simulink model "test00_mdl"  (R2024a)
settings: Solver=ode1  StartTime=0.0  StopTime=Inf  FixedStep=0.001  RelTol=1e-3
PostLoadFcn:
  | , if any(exist('dsrtsu_mdlpostloadfcn', 'file') ~= 0), dsrtsu_mdlpostloadfcn('Execute', bdroot); end,
InitFcn:
  | , if any(exist('rtifpga_mdlclblib', 'file') ~= 0), rtifpga_mdlclblib('Init', bdroot); end,
libraries: rti1401lib_dio_type3 x2, rti1401lib_adc_type4 x1, rti1401lib_II_base x1
Description:
  | Standard RTI1401 template.
  | Supported MATLAB version:  R2024a.
settings Model: Tag=RTI1401  DSRTSU_INTERNAL_RTI_VER=640  DSRTSU_INTERNAL_RTI_TYPE=rti1401  RTICANMMDATA=struct('GeneralSetupData',struct('modelroot','C:\Users\VM-User\Desktop\MigrationScripts','generalsettings',struct('filesettings',struct('destfolder',struct('Name','RTICANMM_FILES','Check',1),'buildfolder',struct('Name','.','Check',1),'AbsDestfolder',struct('Name','C:\Users\VM-User\Desktop\MigrationScripts\RTICANMM_FILES'),'AbsBuildfolder',struct('Name','C:\Users\VM-User\Desktop\MigrationScripts'))),'options',struct('addpaths',1,'rmpaths',1,'addtrcexclusion',true,'cannavigator',struct('checkmonitoring',0),'show_usrtrc',0,'use_usrtrc',0),'advanced',struct('options',ones(1,100)),'MPSetup',{{}},'RTI',struct('Type','RTI1401','Ver','7.17','Date','02-Nov-2021'),'modelname','','block','untitled'))  DSRTSU_INTERNAL_RTIFPGA=210  DSRTSU_INTERNAL_RTISTBM_VER=24.1  Creator=carpc  LastModifiedBy=carpc
settings SolverCC: AlgebraicLoopSolver=TrustRegion
settings DataIOCC: ReturnWorkspaceOutputs=off
settings OptimizationCC: BlockReduction=off  OptimizeBlockIOStorage=off  BufferReuse=off  ReuseModelBlockBuffer=off  GlobalBufferReuse=off  ExpressionFolding=off  LocalBlockOutputs=off  OptimizeDataStoreBuffers=off  BusAssignmentInplaceUpdate=off
settings DebuggingCC: UnconnectedInputMsg=warning  UnconnectedOutputMsg=warning  UnconnectedLineMsg=warning  PregeneratedLibrarySubsystemCodeDiagnostic=none  ArithmeticOperatorsInVariantConditions=warning
settings HardwareCC: ProdBitPerPointer=32  ProdBitPerSizeT=32  ProdBitPerPtrDiffT=32  ProdLargestAtomicInteger=Integer  ProdEndianess=BigEndian  ProdWordSize=32  ProdLongLongMode=on  ProdHWDeviceType=Custom Processor->Custom  TargetIntDivRoundTo=Zero  TargetEndianess=BigEndian  TargetHWDeviceType=Custom Processor->Custom
settings ModelReferenceCC: EnableRefExpFcnMdlSchedulingChecks=on  EnableParallelModelReferenceBuilds=on  ParallelModelReferenceMATLABWorkerInit=Load Top Model
settings SFSimCC: SimUseLocalCustomCode=off  MATLABDynamicMemAlloc=off  CustomCodeUndefinedFunction=UseInterfaceOnly
settings RTWCC: Description=dSPACE DS1401 Hardware Platform  SystemTargetFile=rti1401.tlc  MakeCommand=make_rti  TemplateMakefile=rti1401.tmf  RTWUseLocalCustomCode=off  GPUComputeCapability=3.5  DLArmComputeVersion=19.05
settings CodeAppCC: StateflowObjectComments=on
settings STFCustomTargetCC: TargetLangStandard=C89/C90 (ANSI)  ParMdlRefBuildCompliant=on  GRTInterface=off  UseToolchainInfoCompliant=off  SystemTargetFile=rti1401.tlc
settings GRTTargetCC: TargetLangStandard=C89/C90 (ANSI)  CompOptLevelCompliant=off  ConcurrentExecutionCompliant=off  CombineOutputUpdateFcns=off  MatFileLogging=off  CPPClassGenCompliant=off  UseToolchainInfoCompliant=off
settings ConfigComp: CovMetricSettings=dswe

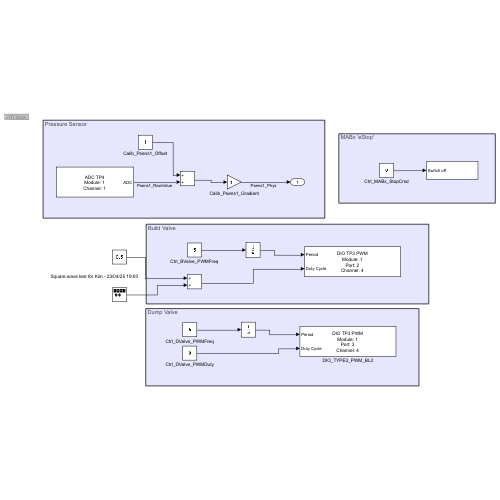
[thumbnail: Simulink's stored preview of the top-level diagram]
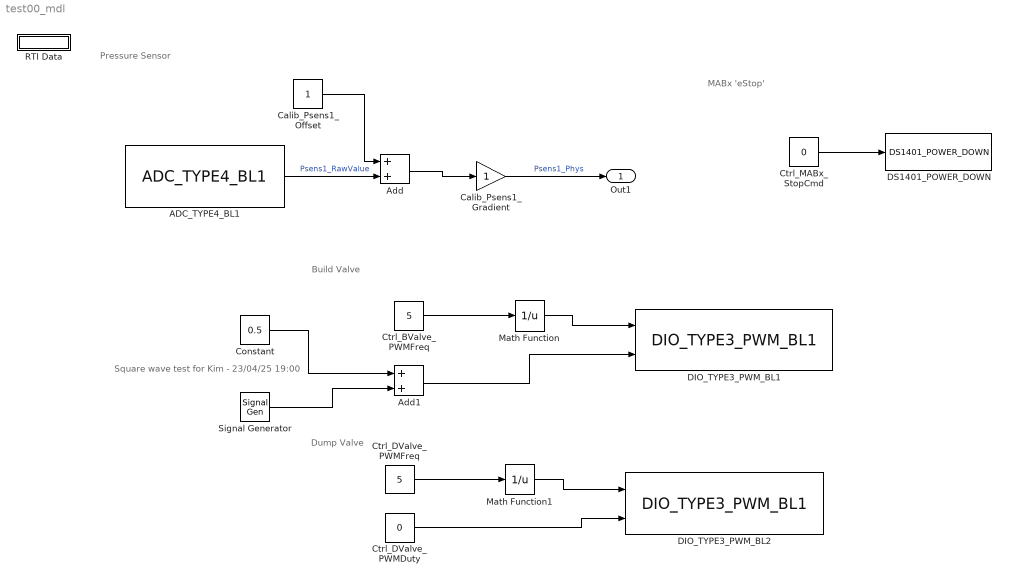
== system test00_mdl ==
  note: Square wave test for Kim - 23/04/25 19:00
  note: MABx 'eStop'
  note: Pressure Sensor
  note: Build Valve
  note: Dump Valve
  ADC_TYPE4_BL1 : rti1401lib_adc_type4/ADC_TYPE4_BL1  DSProperties=struct('RTI',struct('Version',uint32(2),'BlockType',struct('isSLSource',uint8(1),'isSLSink',uint8(1),'isHWSource',uint8(0),'isHWSink',uint8(1),'isSetup',uint8(0),'isInline',uint8(1),'isNonInline',uint8(0),'isInterrupt',uint8(0),'isChannelwise',uint8(1)),'IOBoardType',{{'DS1401','STD','ADCT4'}},'UnitType','ADC','Identifier','ADC','DialogType','ML','BlockSet','NONE','SlaveProcessor','NONE'))  RTIBlockInterface=struct('InputPortsActive',0,'InputPortsWidth',int32(1),'InputPortsDataType',{{'SS_BOOLEAN'}},'InputPortsName',{{'Continue'}},'OutputPortsActive',[1 0],'OutputPortsWidth',int32([1 1]),'OutputPortsDataType',{{'SS_DOUBLE','SS_UINT8'}},'OutputPortsName',{{'ADC','Status'}},'DialogFcn','rti1401stdadct4adcgui','SampleTime',{{-1}},'InitLevel',3,'IconTransparency','on','BlockDisplay',{{['ADC TP4\nModule: 1\nChannel: 1'],'center'}},'BlockName',struct('Token',{{'ADC_TYPE4_BL1'}}))  RTIBlockParameters=struct('ADCSWStartDisable',{{0,'OFF',[0 1]}},'ModuleNo',{{1,'OFF',[1 16]}},'ChannelNo',{{1,'OFF',[1 16]}},'ConversionMode',{{1,'OFF',[1 2]}},'SampleMode',{{1,'OFF',[1 2]}},'TriggerSource',{{1,'OFF',[1 5]}},'EdgePolarity',{{1,'OFF',[1 2]}},'ConversionTriggerSource',{{2,'OFF',[1 6]}},'ConversionEdgePolarity',{{1,'OFF',[1 2]}},'ConversionPeriod',{{1e-6,'OFF',[]}},'ConversionPeriodCheck',{{0,'OFF',[]}},'BurstTriggerSource',{{1,'OFF',[1 6]}},'BurstEdgePolarity',{{1,'OFF',[1 2]}},'BurstSize',{{10,'OFF',[]}},'BurstSizeCheck',{{0,'OFF',[]}},'DataSetOffset',{{0,'OFF',[]}},'DataSetOffsetCheck',{{0,'OFF',[]}},'DataSetLength',{{1,'OFF',[]}},'DataSetLengthCheck',{{0,'OFF',[]}},'ReadMode',{{1,'OFF',[1 2]}},'SampleTime',{{-1,'OFF',[-1 inf]}},'SampleTimeCheck',{{1,'OFF',[]}},'StatusPortEnable',{{0,'OFF',[0 1]}},'VoltageRange',{{1,'OFF',[1 2]}},'TLCFileName',{{'rti1401adc_t4_adc','OFF',[]}})  RTISFcnParameters=struct('ADCSWStartDisable','int32','ModuleNo','int32','ChannelNo','int16','ConversionMode','int16','SampleMode','int16','TriggerSource','int16','EdgePolarity','int16','ConversionTriggerSource','int16','ConversionEdgePolarity','int16','ConversionPeriod','double','BurstTriggerSource','int16','BurstEdgePolarity','int16','BurstSize','int16','DataSetOffset','int16','DataSetLength','int16','ReadMode','int16','SampleTime','double','StatusPortEnable','int16','VoltageRange','int16','TLCFileName','char')  RTIBlockParaDefault=struct('ADCSWStartDisable',0,'ModuleNo',1,'ChannelNo',1,'ConversionMode',1,'SampleMode',1,'TriggerSource',1,'EdgePolarity',1,'ConversionTriggerSource',2,'ConversionEdgePolarity',1,'ConversionPeriod',1e-6,'ConversionPeriodCheck',0,'BurstTriggerSource',1,'BurstEdgePolarity',1,'BurstSize',10,'BurstSizeCheck',0,'DataSetOffset',0,'DataSetOffsetCheck',0,'DataSetLength',1,'DataSetLengthCheck',0,'ReadMode',1,'SampleTime',-1,'SampleTimeCheck',1,'StatusPortEnable',0,'VoltageRange',1,'TLCFileName','rti1401adc_t4_adc')
  Add : Sum
  Add1 : Sum
  Calib_Psens1_Gradient : Gain
  Calib_Psens1_Offset : Constant
  Constant : Constant  Value=0.5
  Ctrl_BValve_PWMFreq : Constant  Value=5
  Ctrl_DValve_PWMDuty : Constant  Value=0
  Ctrl_DValve_PWMFreq : Constant  Value=5
  Ctrl_MABx_StopCmd : Constant  Value=0
  DIO_TYPE3_PWM_BL1 : rti1401lib_dio_type3/DIO_TYPE3_PWM_BL1  DSProperties=struct('RTI',struct('Version',uint32(2),'BlockType',struct('isSLSource',uint8(0),'isSLSink',uint8(1),'isHWSource',uint8(0),'isHWSink',uint8(1),'isSetup',uint8(0),'isInline',uint8(1),'isNonInline',uint8(0),'isInterrupt',uint8(0),'isChannelwise',uint8(1)),'IOBoardType',{{'DS1401','STD','DIOT3'}},'UnitType','PWM','Identifier','PWM','DialogType','ML','BlockSet','NONE','SlaveProcessor','NONE'))  RTIBlockInterface=struct('InputPortsWidth',int32([1 1]),'InputPortsActive',[1 1],'InputPortsName',{{'Period',['Duty Cycle']}},'BlockDisplay',{{['DIO TP3 PWM\nModule: 1\nPort: 2\nChannel: 4'],'center'}},'IconTransparency','on','InitLevel',3,'DialogFcn','rti1401stddiot3pwmgui','BlockName',struct('Token',{{'DIO_TYPE3_PWM_BL1'}}))  RTIBlockParameters=struct('ModuleNo',{{1,'OFF',[1 16]}},'PortNo',{{2,'OFF',[1 3]}},'ChannelNo',{{4,'OFF',[1 16]}},'SupplyRailsCh',{{[1 1],'OFF',[0 1 0 1]}},'UpdateMode',{{1,'ON',[1 2]}},'PeriodRange',{{7,'OFF',[1 16]}},'DutyCycleInit',{{'0','OFF',[0 1]}},'PeriodInit',{{'5e-05','OFF',[]}},'TerminationMode',{{0,'OFF',[0 1]}},'OutputTermValidate',{{0,'OFF',[0 1]}},'OutputTermBuildCheck',{{0,'OFF',[]}},'DutyCycleTerm',{{'0','OFF',[0 1]}},'PeriodTerm',{{'5e-05','OFF',[]}},'TLCFileName',{{'rti1401dio_t3_pwm','OFF',[]}},'EnableInterrupt',{{0,'OFF',[0 1]}},'TriggerEdgeType',{{1,'OFF',[1 3]}})  RTISFcnParameters=struct('ModuleNo','int32','PortNo','int16','ChannelNo','int16','SupplyRailsCh','int16','UpdateMode','int16','PeriodRange','int16','DutyCycleInit','double','PeriodInit','double','TerminationMode','int16','OutputTermValidate','int16','DutyCycleTerm','double','PeriodTerm','double','TLCFileName','char','EnableInterrupt','int16','TriggerEdgeType','int32')  RTIBlockParaDefault=struct('ModuleNo',1,'PortNo',1,'ChannelNo',1,'SupplyRailsCh',[1 1],'UpdateMode',1,'PeriodRange',7,'DutyCycleInit',0,'PeriodInit',5e-5,'TerminationMode',0,'OutputTermValidate',0,'OutputTermBuildCheck',0,'DutyCycleTerm',0,'PeriodTerm',5e-5,'TLCFileName','rti1401dio_t3_pwm','EnableInterrupt',0,'TriggerEdgeType',1)
  DIO_TYPE3_PWM_BL2 : rti1401lib_dio_type3/DIO_TYPE3_PWM_BL1  DSProperties=struct('RTI',struct('Version',uint32(2),'BlockType',struct('isSLSource',uint8(0),'isSLSink',uint8(1),'isHWSource',uint8(0),'isHWSink',uint8(1),'isSetup',uint8(0),'isInline',uint8(1),'isNonInline',uint8(0),'isInterrupt',uint8(0),'isChannelwise',uint8(1)),'IOBoardType',{{'DS1401','STD','DIOT3'}},'UnitType','PWM','Identifier','PWM','DialogType','ML','BlockSet','NONE','SlaveProcessor','NONE'))  RTIBlockInterface=struct('InputPortsWidth',int32([1 1]),'InputPortsActive',[1 1],'InputPortsName',{{'Period',['Duty Cycle']}},'BlockDisplay',{{['DIO TP3 PWM\nModule: 1\nPort: 3\nChannel: 4'],'center'}},'IconTransparency','on','InitLevel',3,'DialogFcn','rti1401stddiot3pwmgui','BlockName',struct('Token',{{'DIO_TYPE3_PWM_BL1'}}))  RTIBlockParameters=struct('ModuleNo',{{1,'OFF',[1 16]}},'PortNo',{{3,'OFF',[1 3]}},'ChannelNo',{{4,'OFF',[1 8]}},'SupplyRailsCh',{{[1 1],'OFF',[0 1 0 1]}},'UpdateMode',{{1,'ON',[1 2]}},'PeriodRange',{{7,'OFF',[1 16]}},'DutyCycleInit',{{'0','OFF',[0 1]}},'PeriodInit',{{'5e-05','OFF',[]}},'TerminationMode',{{0,'OFF',[0 1]}},'OutputTermValidate',{{0,'OFF',[0 1]}},'OutputTermBuildCheck',{{0,'OFF',[]}},'DutyCycleTerm',{{'0','OFF',[0 1]}},'PeriodTerm',{{'5e-05','OFF',[]}},'TLCFileName',{{'rti1401dio_t3_pwm','OFF',[]}},'EnableInterrupt',{{0,'OFF',[0 1]}},'TriggerEdgeType',{{1,'OFF',[1 3]}})  RTISFcnParameters=struct('ModuleNo','int32','PortNo','int16','ChannelNo','int16','SupplyRailsCh','int16','UpdateMode','int16','PeriodRange','int16','DutyCycleInit','double','PeriodInit','double','TerminationMode','int16','OutputTermValidate','int16','DutyCycleTerm','double','PeriodTerm','double','TLCFileName','char','EnableInterrupt','int16','TriggerEdgeType','int32')  RTIBlockParaDefault=struct('ModuleNo',1,'PortNo',1,'ChannelNo',1,'SupplyRailsCh',[1 1],'UpdateMode',1,'PeriodRange',7,'DutyCycleInit',0,'PeriodInit',5e-5,'TerminationMode',0,'OutputTermValidate',0,'OutputTermBuildCheck',0,'DutyCycleTerm',0,'PeriodTerm',5e-5,'TLCFileName','rti1401dio_t3_pwm','EnableInterrupt',0,'TriggerEdgeType',1)
  DS1401_POWER_DOWN : rti1401lib_II_base/DS1401_POWER_DOWN  Reserved1=[]  Reserved2=[]  Reserved3=[]  Reserved4=[]  DSProperties=struct('RTI',struct('Version',uint32(1),'BlockType',struct('isSLSource',uint8(0),'isSLSink',uint8(1),'isHWSource',uint8(0),'isHWSink',uint8(0),'isSetup',uint8(0),'isInline',uint8(0),'isNonInline',uint8(1),'isInterrupt',uint8(0),'isChannelwise',uint8(0)),'IOBoardType',{{'DS1401','BASE'}},'UnitType','POWER','Identifier','POWERDOWN','DialogType','ML','BlockSet','NONE','SlaveProcessor','NONE'))  RTIBlockInterface="struct('InputPortsActive',1,'InputPortsWidth',int32(1),'InputPortsName',{{['Switch off']}},'IconTransparency','on','DialogFcn','gui1401powerdown','InitLevel',1,'BlockName',struct('Token',{{'DS1401_POWER_DOWN'}}),'MaskDescription',['If the hardware input \"Remote In\" is switched off, the MicroAutoBox powers down.'])"  RTIBlockParameters=struct('TLCFileName',{{'rti1401powerdown','OFF',[]}})  RTISFcnParameters=struct('TLCFileName','char')  RTIBlockParaDefault=struct('TLCFileName','rti1401powerdown')
  Math Function : Math  Operator=reciprocal
  Math Function1 : Math  Operator=reciprocal
  RTI Data : Subsystem  Tag=struct('RTIDataServer',struct('RTIDataServerVs','2','RTIModelDescription','struct(''main'',''test00_mdl'',''sub'','''',''isMp'',0)'))  LoadFcn="if exist('rtidc'), try,  rtidc('DataHostBlockClbLoad', gcbh); catch, disp(['Warning: ''LoadFcn'' for RTI Data block failed: ' lasterr]); end, end,"  mask(RTI_DATA_HOST){}
      mask help:
      | RTI Data Block.
      | This block is used by RTI to store internal model-dependent data.
      | Please keep this block on the root level of the model. Deleting this block will result in data loss.
      |
      | NEVER DELETE OR COPY THIS BLOCK!
      settings: CopyFcn="if exist('rtidc'), try,  rtidc('DataHostBlockClbCopy', gcbh); catch, disp(['Warning: ''CopyFcn'' for RTI Data block failed: ' lasterr]); end, end,"  DeleteFcn="if exist('rtidc'), try,  rtidc('DataHostBlockClbDelete', gcbh); catch, disp(['Warning: ''DeleteFcn'' for RTI Data block failed: ' lasterr]); end, end,"  ModelCloseFcn="if exist('rtidc'), try,  rtidc('DataHostBlockClbModelClose', gcbh); catch, disp(['Warning: ''ModelCloseFcn'' for RTI Data block failed: ' lasterr]); end, end,"  PreSaveFcn="if exist('rtidc'), try,  rtidc('DataHostBlockClbPreSave', gcbh); catch, disp(['Warning: ''PreSaveFcn'' for RTI Data block failed: ' lasterr]); end, end,"  PostSaveFcn="if exist('rtidc'), try,  rtidc('DataHostBlockClbPostSave', gcbh); catch, disp(['Warning: ''PostSaveFcn'' for RTI Data block failed: ' lasterr]); end, end,"  NameChangeFcn="if exist('rtidc'), try,  rtidc('DataHostBlockClbNameChange', gcbh); catch, disp(['Warning: ''NameChangeFcn'' for RTI Data block failed: ' lasterr]); end, end,"
      mask Help:
      | RTI Data Block.
      | This block is used by RTI to store internal model-dependent data.
      | Please keep this block on the root level of the model. Deleting this block will result in data loss.
      | 
      | NEVER DELETE OR COPY THIS BLOCK!
      mask Display:
      | text(0.5, 0.5, 'RTI Data', 'HorizontalAlignment', 'center');
      | plot([1 0]);
  Signal Generator : SignalGenerator  WaveForm=square  Amplitude=0.5  Units=rad/sec
  Out1 : Outport
  wires:
  Ctrl_MABx_StopCmd/1 -> DS1401_POWER_DOWN/1
  Add/1 -> Calib_Psens1_Gradient/1
  Calib_Psens1_Gradient/1 -> Out1/1  "Psens1_Phys"
  Calib_Psens1_Offset/1 -> Add/1
  ADC_TYPE4_BL1/1 -> Add/2  "Psens1_RawValue"
  Math Function/1 -> DIO_TYPE3_PWM_BL1/1
  Signal Generator/1 -> Add1/2
  Ctrl_BValve_PWMFreq/1 -> Math Function/1
  Ctrl_DValve_PWMFreq/1 -> Math Function1/1
  Math Function1/1 -> DIO_TYPE3_PWM_BL2/1
  Ctrl_DValve_PWMDuty/1 -> DIO_TYPE3_PWM_BL2/2
  Add1/1 -> DIO_TYPE3_PWM_BL1/2
  Constant/1 -> Add1/1

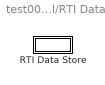
== system test00_mdl/RTI Data ==
  RTI Data Store : Subsystem  Tag="struct('public',struct('sub',struct('name',{{'test00_mdl'}},'data',{{struct('TH',struct('thTaskInfo',struct('taskType',{'TIMER','HWINT','TMRINT','SWINT','GLINT'},'tasksNumOf',{1,0,0,0,0},'srcIds',{{'TIMERA'},{},{},{},{}},'taskNames',{{['Timer Task 1']},{},{},{},{}})),'th_tc',struct('dataType','TASK','taskGroupId','','taskGroupList',{{}},'taskSchedulingPolicy','FCFS','taskType','TIMER','blkh',-1,'srcId','TIMERA','srcSgnName',['Timer A interrupt'],'srcCpuName','','taskName',['Timer Task 1  [0.001] s'],'taskNameDisplayExt','','smplTime',0.001,'smplTimeOffs',0,'hasFixedPriority',0,'priority',1,'hasFixedOvc',0,'ovcType',1,'ovcMax',1),'tc_th',struct('dataType','TASK','taskGroupId','','taskGroupList',{{}},'taskSchedulingPolicy','FCFS','taskType','TIMER','blkh',-1,'srcId','TIMERA','srcSgnName',['Timer A interrupt'],'srcCpuName','','taskName',['Timer Task 1  [0.001] s'],'taskNameDisplayExt','','smplTime',0.001,'smplTimeOffs',0,'hasFixedPriority',0,'priority',1,'hasFixedOvc',0,'ovcType',1,'ovcMax',1))}})),'private',struct('version',struct('dsVer',uint32(2)),'access',struct('type','Model','isPerm',1)))"  mask(RTI_DATA_STORE){}
      mask help:
      | RTI Data Store Block. This block is used by RTI to store internal model dependent data. Deleting this block will result in data loss.
      |
      | NEVER DELETE, COPY, OR MODIFY THIS BLOCK!
      mask Help:
      | RTI Data Store Block. This block is used by RTI to store internal model dependent data. Deleting this block will result in data loss.
      | 
      | NEVER DELETE, COPY, OR MODIFY THIS BLOCK!
      mask Display: text(0.5, 0.5, ' ', 'HorizontalAlignment', 'center');

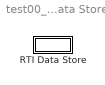
== system test00_mdl/RTI Data/RTI Data Store ==
  RTI Data Store : Subsystem  mask(RTI_DATA_STORE){}
      mask help:
      | RTI Data Store Block. This block is used by RTI to store internal model dependent data. Deleting this block will result in data loss.
      |
      | NEVER DELETE, COPY, OR MODIFY THIS BLOCK!
      mask Help:
      | RTI Data Store Block. This block is used by RTI to store internal model dependent data. Deleting this block will result in data loss.
      | 
      | NEVER DELETE, COPY, OR MODIFY THIS BLOCK!
      mask Display: text(0.5, 0.5, ' ', 'HorizontalAlignment', 'center');

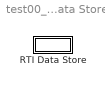
== system test00_mdl/RTI Data/RTI Data Store/RTI Data Store ==
  RTI Data Store : Subsystem  mask(RTI_DATA_STORE){}
      mask help:
      | RTI Data Store Block. This block is used by RTI to store internal model dependent data. Deleting this block will result in data loss.
      |
      | NEVER DELETE, COPY, OR MODIFY THIS BLOCK!
      mask Help:
      | RTI Data Store Block. This block is used by RTI to store internal model dependent data. Deleting this block will result in data loss.
      | 
      | NEVER DELETE, COPY, OR MODIFY THIS BLOCK!
      mask Display: text(0.5, 0.5, ' ', 'HorizontalAlignment', 'center');

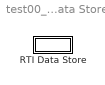
== system test00_mdl/RTI Data/RTI Data Store/RTI Data Store/RTI Data Store ==
  RTI Data Store : Subsystem  mask(RTI_DATA_STORE){}
      mask help:
      | RTI Data Store Block. This block is used by RTI to store internal model dependent data. Deleting this block will result in data loss.
      |
      | NEVER DELETE, COPY, OR MODIFY THIS BLOCK!
      mask Help:
      | RTI Data Store Block. This block is used by RTI to store internal model dependent data. Deleting this block will result in data loss.
      | 
      | NEVER DELETE, COPY, OR MODIFY THIS BLOCK!
      mask Display: text(0.5, 0.5, ' ', 'HorizontalAlignment', 'center');

== system test00_mdl/RTI Data/RTI Data Store/RTI Data Store/RTI Data Store/RTI Data Store ==
